simulink model "FaultModel"  (R2022b)
settings: Solver=VariableStepAuto  StartTime=0.0  StopTime=0.05  RelTol=1e-3
undefined symbols (not defined in the file or in its folder): D1, Delta
libraries: spsThreePhaseTransformerTwoWindingsLib x97, spsThreePhaseParallelRLCLoadLib x86, spsDistributedParametersLineLib x60, spsThreePhaseVIMeasurementLib x34, spsThreePhaseSourceLib x30, spsSeriesRLCBranchLib x3, spsGroundLib x2, spsCurrentMeasurementLib x1, spsThreePhaseFaultLib x1, spsVoltageMeasurementLib x1, spspowerguiLib x1
(part 4 of 4)

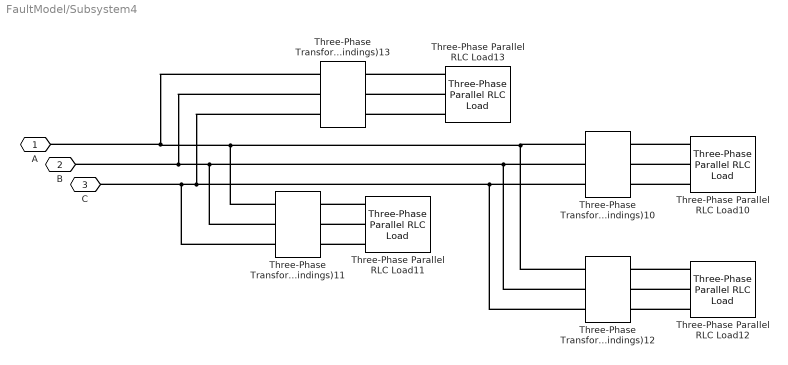
== system FaultModel/Subsystem4 ==
  Three-Phase Parallel RLC Load10 : spsThreePhaseParallelRLCLoadLib/Three-Phase Parallel RLC Load  LConnTagsString=A|B|C  Configuration=Y (grounded)  NominalVoltage=33e3  Vabc=[1e3 1e3 1e3]  Vabcp=[1e3 1e3 1e3]  NominalFrequency=50  UnbalancedPower=off  ActivePower=32.8e6  InductivePower=100  CapacitivePower=100  Pabc=[10e3 9e3 11e3]  QLabc=[100 90 110]  QCabc=[100 90 110]  Pabcp=[10e3 9e3 11e3]  QLabcp=[100 90 110]  QCabcp=[100 90 110]  Measurements=None  LoadType=constant Z
  Three-Phase Parallel RLC Load11 : spsThreePhaseParallelRLCLoadLib/Three-Phase Parallel RLC Load  LConnTagsString=A|B|C  Configuration=Y (grounded)  NominalVoltage=33e3  Vabc=[1e3 1e3 1e3]  Vabcp=[1e3 1e3 1e3]  NominalFrequency=50  UnbalancedPower=off  ActivePower=32.8e6  InductivePower=100  CapacitivePower=100  Pabc=[10e3 9e3 11e3]  QLabc=[100 90 110]  QCabc=[100 90 110]  Pabcp=[10e3 9e3 11e3]  QLabcp=[100 90 110]  QCabcp=[100 90 110]  Measurements=None  LoadType=constant Z
  Three-Phase Parallel RLC Load12 : spsThreePhaseParallelRLCLoadLib/Three-Phase Parallel RLC Load  LConnTagsString=A|B|C  Configuration=Y (grounded)  NominalVoltage=33e3  Vabc=[1e3 1e3 1e3]  Vabcp=[1e3 1e3 1e3]  NominalFrequency=50  UnbalancedPower=off  ActivePower=60e6  InductivePower=100  CapacitivePower=100  Pabc=[10e3 9e3 11e3]  QLabc=[100 90 110]  QCabc=[100 90 110]  Pabcp=[10e3 9e3 11e3]  QLabcp=[100 90 110]  QCabcp=[100 90 110]  Measurements=None  LoadType=constant Z
  Three-Phase Parallel RLC Load13 : spsThreePhaseParallelRLCLoadLib/Three-Phase Parallel RLC Load  LConnTagsString=A|B|C  Configuration=Y (grounded)  NominalVoltage=33e3  Vabc=[1e3 1e3 1e3]  Vabcp=[1e3 1e3 1e3]  NominalFrequency=50  UnbalancedPower=off  ActivePower=40e6  InductivePower=100  CapacitivePower=100  Pabc=[10e3 9e3 11e3]  QLabc=[100 90 110]  QCabc=[100 90 110]  Pabcp=[10e3 9e3 11e3]  QLabcp=[100 90 110]  QCabcp=[100 90 110]  Measurements=None  LoadType=constant Z
  Three-Phase Transformer (Two Windings)10 : spsThreePhaseTransformerTwoWindingsLib/Three-Phase Transformer (Two Windings)  Winding1Connection=Delta (D1)  Winding2Connection=Yg  CoreType=Three single-phase transformers  SetSaturation=off  Hysteresis=off  DataFile='hysteresis'  SetInitialFlux=off  Measurements=None  UNITS=pu  NominalPower=[ 41e6 , 50 ]  Winding1=[ 132e3 , 0.002 , 0.08 ]  Winding2=[ 33e3 , 0.002 , 0.08 ]  Rm=500  Lm=500  L0=0.5  Saturation=[ 0,0 ; 0.0024,1.2 ; 1.0,1.52 ]  InitialFluxes=[ 0.8 , -0.8 , 0.7 ]  BreakLoop=off  DiscreteSolver=Trapezoidal iterative  DataType=off  TransfoNumber=1
  Three-Phase Transformer (Two Windings)11 : spsThreePhaseTransformerTwoWindingsLib/Three-Phase Transformer (Two Windings)  Winding1Connection=Delta (D1)  Winding2Connection=Yg  CoreType=Three single-phase transformers  SetSaturation=off  Hysteresis=off  DataFile='hysteresis'  SetInitialFlux=off  Measurements=None  UNITS=pu  NominalPower=[ 41e6 , 50 ]  Winding1=[ 132e3 , 0.002 , 0.08 ]  Winding2=[ 33e3 , 0.002 , 0.08 ]  Rm=500  Lm=500  L0=0.5  Saturation=[ 0,0 ; 0.0024,1.2 ; 1.0,1.52 ]  InitialFluxes=[ 0.8 , -0.8 , 0.7 ]  BreakLoop=off  DiscreteSolver=Trapezoidal iterative  DataType=off  TransfoNumber=1
  Three-Phase Transformer (Two Windings)12 : spsThreePhaseTransformerTwoWindingsLib/Three-Phase Transformer (Two Windings)  Winding1Connection=Delta (D1)  Winding2Connection=Yg  CoreType=Three single-phase transformers  SetSaturation=off  Hysteresis=off  DataFile='hysteresis'  SetInitialFlux=off  Measurements=None  UNITS=pu  NominalPower=[ 75e6 , 50 ]  Winding1=[ 132e3 , 0.002 , 0.08 ]  Winding2=[ 33e3 , 0.002 , 0.08 ]  Rm=500  Lm=500  L0=0.5  Saturation=[ 0,0 ; 0.0024,1.2 ; 1.0,1.52 ]  InitialFluxes=[ 0.8 , -0.8 , 0.7 ]  BreakLoop=off  DiscreteSolver=Trapezoidal iterative  DataType=off  TransfoNumber=1
  Three-Phase Transformer (Two Windings)13 : spsThreePhaseTransformerTwoWindingsLib/Three-Phase Transformer (Two Windings)  Winding1Connection=Delta (D1)  Winding2Connection=Yg  CoreType=Three single-phase transformers  SetSaturation=off  Hysteresis=off  DataFile='hysteresis'  SetInitialFlux=off  Measurements=None  UNITS=pu  NominalPower=[50e6 , 50 ]  Winding1=[ 132e3 , 0.002 , 0.08 ]  Winding2=[ 33e3 , 0.002 , 0.08 ]  Rm=500  Lm=500  L0=0.5  Saturation=[ 0,0 ; 0.0024,1.2 ; 1.0,1.52 ]  InitialFluxes=[ 0.8 , -0.8 , 0.7 ]  BreakLoop=off  DiscreteSolver=Trapezoidal iterative  DataType=off  TransfoNumber=1
  A : PMIOPort  Side=Left
  B : PMIOPort  Port=2  Side=Left
  C : PMIOPort  Port=3  Side=Left
  connections:
  Three-Phase Parallel RLC Load10/LConn3 -- Three-Phase Transformer (Two Windings)10/RConn3
  Three-Phase Parallel RLC Load10/LConn2 -- Three-Phase Transformer (Two Windings)10/RConn2
  Three-Phase Parallel RLC Load13/LConn3 -- Three-Phase Transformer (Two Windings)13/RConn3
  Three-Phase Parallel RLC Load11/LConn3 -- Three-Phase Transformer (Two Windings)11/RConn3
  Three-Phase Transformer (Two Windings)13/LConn2 -- B/RConn1 -- Three-Phase Transformer (Two Windings)12/LConn2 -- Three-Phase Transformer (Two Windings)10/LConn2 -- Three-Phase Transformer (Two Windings)11/LConn2
  Three-Phase Parallel RLC Load12/LConn2 -- Three-Phase Transformer (Two Windings)12/RConn2
  Three-Phase Transformer (Two Windings)13/LConn1 -- Three-Phase Transformer (Two Windings)11/LConn1 -- Three-Phase Transformer (Two Windings)12/LConn1 -- Three-Phase Transformer (Two Windings)10/LConn1 -- A/RConn1
  Three-Phase Parallel RLC Load13/LConn2 -- Three-Phase Transformer (Two Windings)13/RConn2
  Three-Phase Parallel RLC Load12/LConn1 -- Three-Phase Transformer (Two Windings)12/RConn1
  Three-Phase Parallel RLC Load11/LConn2 -- Three-Phase Transformer (Two Windings)11/RConn2
  Three-Phase Parallel RLC Load11/LConn1 -- Three-Phase Transformer (Two Windings)11/RConn1
  Three-Phase Transformer (Two Windings)12/LConn3 -- C/RConn1 -- Three-Phase Transformer (Two Windings)11/LConn3 -- Three-Phase Transformer (Two Windings)13/LConn3 -- Three-Phase Transformer (Two Windings)10/LConn3
  Three-Phase Parallel RLC Load13/LConn1 -- Three-Phase Transformer (Two Windings)13/RConn1
  Three-Phase Parallel RLC Load12/LConn3 -- Three-Phase Transformer (Two Windings)12/RConn3
  Three-Phase Parallel RLC Load10/LConn1 -- Three-Phase Transformer (Two Windings)10/RConn1

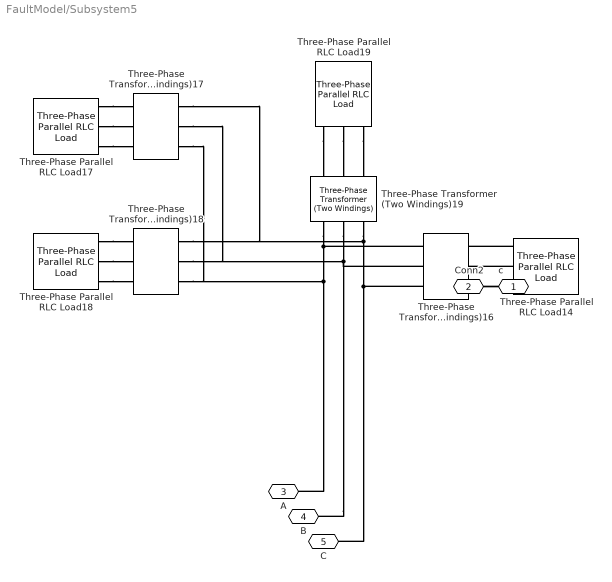
== system FaultModel/Subsystem5 ==
  Three-Phase Parallel RLC Load14 : spsThreePhaseParallelRLCLoadLib/Three-Phase Parallel RLC Load  LConnTagsString=A|B|C  Configuration=Y (grounded)  NominalVoltage=33e3  Vabc=[1e3 1e3 1e3]  Vabcp=[1e3 1e3 1e3]  NominalFrequency=50  UnbalancedPower=off  ActivePower=32.8e6  InductivePower=100  CapacitivePower=100  Pabc=[10e3 9e3 11e3]  QLabc=[100 90 110]  QCabc=[100 90 110]  Pabcp=[10e3 9e3 11e3]  QLabcp=[100 90 110]  QCabcp=[100 90 110]  Measurements=None  LoadType=constant Z
  Three-Phase Parallel RLC Load17 : spsThreePhaseParallelRLCLoadLib/Three-Phase Parallel RLC Load  LConnTagsString=A|B|C  Configuration=Y (grounded)  NominalVoltage=33e3  Vabc=[1e3 1e3 1e3]  Vabcp=[1e3 1e3 1e3]  NominalFrequency=50  UnbalancedPower=off  ActivePower=32.8e6  InductivePower=100  CapacitivePower=100  Pabc=[10e3 9e3 11e3]  QLabc=[100 90 110]  QCabc=[100 90 110]  Pabcp=[10e3 9e3 11e3]  QLabcp=[100 90 110]  QCabcp=[100 90 110]  Measurements=None  LoadType=constant Z
  Three-Phase Parallel RLC Load18 : spsThreePhaseParallelRLCLoadLib/Three-Phase Parallel RLC Load  LConnTagsString=A|B|C  Configuration=Y (grounded)  NominalVoltage=33e3  Vabc=[1e3 1e3 1e3]  Vabcp=[1e3 1e3 1e3]  NominalFrequency=50  UnbalancedPower=off  ActivePower=16e6  InductivePower=100  CapacitivePower=100  Pabc=[10e3 9e3 11e3]  QLabc=[100 90 110]  QCabc=[100 90 110]  Pabcp=[10e3 9e3 11e3]  QLabcp=[100 90 110]  QCabcp=[100 90 110]  Measurements=None  LoadType=constant Z
  Three-Phase Parallel RLC Load19 : spsThreePhaseParallelRLCLoadLib/Three-Phase Parallel RLC Load  LConnTagsString=A|B|C  Configuration=Y (grounded)  NominalVoltage=33e3  Vabc=[1e3 1e3 1e3]  Vabcp=[1e3 1e3 1e3]  NominalFrequency=50  UnbalancedPower=off  ActivePower=16e6  InductivePower=100  CapacitivePower=100  Pabc=[10e3 9e3 11e3]  QLabc=[100 90 110]  QCabc=[100 90 110]  Pabcp=[10e3 9e3 11e3]  QLabcp=[100 90 110]  QCabcp=[100 90 110]  Measurements=None  LoadType=constant Z
  Three-Phase Transformer (Two Windings)16 : spsThreePhaseTransformerTwoWindingsLib/Three-Phase Transformer (Two Windings)  Winding1Connection=Delta (D1)  Winding2Connection=Yg  CoreType=Three single-phase transformers  SetSaturation=off  Hysteresis=off  DataFile='hysteresis'  SetInitialFlux=off  Measurements=None  UNITS=pu  NominalPower=[41e6 , 50 ]  Winding1=[ 132e3 , 0.002 , 0.08 ]  Winding2=[ 33e3 , 0.002 , 0.08 ]  Rm=500  Lm=500  L0=0.5  Saturation=[ 0,0 ; 0.0024,1.2 ; 1.0,1.52 ]  InitialFluxes=[ 0.8 , -0.8 , 0.7 ]  BreakLoop=off  DiscreteSolver=Trapezoidal iterative  DataType=off  TransfoNumber=1
  Three-Phase Transformer (Two Windings)17 : spsThreePhaseTransformerTwoWindingsLib/Three-Phase Transformer (Two Windings)  Winding1Connection=Delta (D1)  Winding2Connection=Yg  CoreType=Three single-phase transformers  SetSaturation=off  Hysteresis=off  DataFile='hysteresis'  SetInitialFlux=off  Measurements=None  UNITS=pu  NominalPower=[41e6 , 50 ]  Winding1=[ 132e3 , 0.002 , 0.08 ]  Winding2=[ 33e3 , 0.002 , 0.08 ]  Rm=500  Lm=500  L0=0.5  Saturation=[ 0,0 ; 0.0024,1.2 ; 1.0,1.52 ]  InitialFluxes=[ 0.8 , -0.8 , 0.7 ]  BreakLoop=off  DiscreteSolver=Trapezoidal iterative  DataType=off  TransfoNumber=1
  Three-Phase Transformer (Two Windings)18 : spsThreePhaseTransformerTwoWindingsLib/Three-Phase Transformer (Two Windings)  Winding1Connection=Delta (D1)  Winding2Connection=Yg  CoreType=Three single-phase transformers  SetSaturation=off  Hysteresis=off  DataFile='hysteresis'  SetInitialFlux=off  Measurements=None  UNITS=pu  NominalPower=[20e6 , 50 ]  Winding1=[ 132e3 , 0.002 , 0.08 ]  Winding2=[ 33e3 , 0.002 , 0.08 ]  Rm=500  Lm=500  L0=0.5  Saturation=[ 0,0 ; 0.0024,1.2 ; 1.0,1.52 ]  InitialFluxes=[ 0.8 , -0.8 , 0.7 ]  BreakLoop=off  DiscreteSolver=Trapezoidal iterative  DataType=off  TransfoNumber=1
  Three-Phase Transformer (Two Windings)19 : spsThreePhaseTransformerTwoWindingsLib/Three-Phase Transformer (Two Windings)  Winding1Connection=Delta (D1)  Winding2Connection=Yg  CoreType=Three single-phase transformers  SetSaturation=off  Hysteresis=off  DataFile='hysteresis'  SetInitialFlux=off  Measurements=None  UNITS=pu  NominalPower=[20e6 , 50 ]  Winding1=[ 132e3 , 0.002 , 0.08 ]  Winding2=[ 33e3 , 0.002 , 0.08 ]  Rm=500  Lm=500  L0=0.5  Saturation=[ 0,0 ; 0.0024,1.2 ; 1.0,1.52 ]  InitialFluxes=[ 0.8 , -0.8 , 0.7 ]  BreakLoop=off  DiscreteSolver=Trapezoidal iterative  DataType=off  TransfoNumber=1
  c : PMIOPort  Side=Right
  Conn2 : PMIOPort  Port=2  Side=Left
  A : PMIOPort  Port=3  Side=Left
  B : PMIOPort  Port=4  Side=Left
  C : PMIOPort  Port=5  Side=Left
  connections:
  Three-Phase Transformer (Two Windings)19/LConn3 -- Three-Phase Transformer (Two Windings)17/LConn3 -- Three-Phase Transformer (Two Windings)18/LConn3 -- C/RConn1 -- Three-Phase Transformer (Two Windings)16/LConn3
  Three-Phase Transformer (Two Windings)19/LConn2 -- Three-Phase Transformer (Two Windings)17/LConn2 -- Three-Phase Transformer (Two Windings)18/LConn2 -- B/RConn1 -- Three-Phase Transformer (Two Windings)16/LConn2
  Three-Phase Transformer (Two Windings)19/LConn1 -- Three-Phase Transformer (Two Windings)16/LConn1 -- A/RConn1 -- Three-Phase Transformer (Two Windings)17/LConn1 -- Three-Phase Transformer (Two Windings)18/LConn1
  Three-Phase Parallel RLC Load17/LConn1 -- Three-Phase Transformer (Two Windings)17/RConn3
  Three-Phase Parallel RLC Load19/LConn1 -- Three-Phase Transformer (Two Windings)19/RConn1
  Three-Phase Parallel RLC Load14/LConn1 -- Three-Phase Transformer (Two Windings)16/RConn1
  Three-Phase Parallel RLC Load18/LConn2 -- Three-Phase Transformer (Two Windings)18/RConn2
  Three-Phase Parallel RLC Load17/LConn2 -- Three-Phase Transformer (Two Windings)17/RConn2
  Three-Phase Parallel RLC Load17/LConn3 -- Three-Phase Transformer (Two Windings)17/RConn1
  Three-Phase Parallel RLC Load19/LConn2 -- Three-Phase Transformer (Two Windings)19/RConn2
  Three-Phase Parallel RLC Load18/LConn1 -- Three-Phase Transformer (Two Windings)18/RConn3
  Three-Phase Parallel RLC Load19/LConn3 -- Three-Phase Transformer (Two Windings)19/RConn3
  Three-Phase Parallel RLC Load14/LConn2 -- Three-Phase Transformer (Two Windings)16/RConn2
  Three-Phase Parallel RLC Load18/LConn3 -- Three-Phase Transformer (Two Windings)18/RConn1
  Three-Phase Transformer (Two Windings)16/RConn3 -- c/RConn1
  Three-Phase Parallel RLC Load14/LConn3 -- Conn2/RConn1

== system FaultModel/Subsystem6 ==
  Three-Phase Parallel RLC Load20 : spsThreePhaseParallelRLCLoadLib/Three-Phase Parallel RLC Load  LConnTagsString=A|B|C  Configuration=Y (grounded)  NominalVoltage=33e3  Vabc=[1e3 1e3 1e3]  Vabcp=[1e3 1e3 1e3]  NominalFrequency=50  UnbalancedPower=off  ActivePower=32.8e6  InductivePower=100  CapacitivePower=100  Pabc=[10e3 9e3 11e3]  QLabc=[100 90 110]  QCabc=[100 90 110]  Pabcp=[10e3 9e3 11e3]  QLabcp=[100 90 110]  QCabcp=[100 90 110]  Measurements=None  LoadType=constant Z
  Three-Phase Parallel RLC Load21 : spsThreePhaseParallelRLCLoadLib/Three-Phase Parallel RLC Load  LConnTagsString=A|B|C  Configuration=Y (grounded)  NominalVoltage=33e3  Vabc=[1e3 1e3 1e3]  Vabcp=[1e3 1e3 1e3]  NominalFrequency=50  UnbalancedPower=off  ActivePower=32.8e6  InductivePower=100  CapacitivePower=100  Pabc=[10e3 9e3 11e3]  QLabc=[100 90 110]  QCabc=[100 90 110]  Pabcp=[10e3 9e3 11e3]  QLabcp=[100 90 110]  QCabcp=[100 90 110]  Measurements=None  LoadType=constant Z
  Three-Phase Parallel RLC Load22 : spsThreePhaseParallelRLCLoadLib/Three-Phase Parallel RLC Load  LConnTagsString=A|B|C  Configuration=Y (grounded)  NominalVoltage=33e3  Vabc=[1e3 1e3 1e3]  Vabcp=[1e3 1e3 1e3]  NominalFrequency=50  UnbalancedPower=off  ActivePower=32.8e6  InductivePower=100  CapacitivePower=100  Pabc=[10e3 9e3 11e3]  QLabc=[100 90 110]  QCabc=[100 90 110]  Pabcp=[10e3 9e3 11e3]  QLabcp=[100 90 110]  QCabcp=[100 90 110]  Measurements=None  LoadType=constant Z
  Three-Phase Transformer (Two Windings)20 : spsThreePhaseTransformerTwoWindingsLib/Three-Phase Transformer (Two Windings)  Winding1Connection=Delta (D1)  Winding2Connection=Yg  CoreType=Three single-phase transformers  SetSaturation=off  Hysteresis=off  DataFile='hysteresis'  SetInitialFlux=off  Measurements=None  UNITS=pu  NominalPower=[41e6 , 50 ]  Winding1=[ 132e3 , 0.002 , 0.08 ]  Winding2=[ 33e3 , 0.002 , 0.08 ]  Rm=500  Lm=500  L0=0.5  Saturation=[ 0,0 ; 0.0024,1.2 ; 1.0,1.52 ]  InitialFluxes=[ 0.8 , -0.8 , 0.7 ]  BreakLoop=off  DiscreteSolver=Trapezoidal iterative  DataType=off  TransfoNumber=1
  Three-Phase Transformer (Two Windings)21 : spsThreePhaseTransformerTwoWindingsLib/Three-Phase Transformer (Two Windings)  Winding1Connection=Delta (D1)  Winding2Connection=Yg  CoreType=Three single-phase transformers  SetSaturation=off  Hysteresis=off  DataFile='hysteresis'  SetInitialFlux=off  Measurements=None  UNITS=pu  NominalPower=[41e6 , 50 ]  Winding1=[ 132e3 , 0.002 , 0.08 ]  Winding2=[ 33e3 , 0.002 , 0.08 ]  Rm=500  Lm=500  L0=0.5  Saturation=[ 0,0 ; 0.0024,1.2 ; 1.0,1.52 ]  InitialFluxes=[ 0.8 , -0.8 , 0.7 ]  BreakLoop=off  DiscreteSolver=Trapezoidal iterative  DataType=off  TransfoNumber=1
  Three-Phase Transformer (Two Windings)22 : spsThreePhaseTransformerTwoWindingsLib/Three-Phase Transformer (Two Windings)  Winding1Connection=Delta (D1)  Winding2Connection=Yg  CoreType=Three single-phase transformers  SetSaturation=off  Hysteresis=off  DataFile='hysteresis'  SetInitialFlux=off  Measurements=None  UNITS=pu  NominalPower=[41e6 , 50 ]  Winding1=[ 132e3 , 0.002 , 0.08 ]  Winding2=[ 33e3 , 0.002 , 0.08 ]  Rm=500  Lm=500  L0=0.5  Saturation=[ 0,0 ; 0.0024,1.2 ; 1.0,1.52 ]  InitialFluxes=[ 0.8 , -0.8 , 0.7 ]  BreakLoop=off  DiscreteSolver=Trapezoidal iterative  DataType=off  TransfoNumber=1
  C : PMIOPort  Side=Left
  B : PMIOPort  Port=2  Side=Left
  A : PMIOPort  Port=3  Side=Left
  connections:
  Three-Phase Parallel RLC Load22/LConn2 -- Three-Phase Transformer (Two Windings)22/RConn2
  Three-Phase Parallel RLC Load22/LConn3 -- Three-Phase Transformer (Two Windings)22/RConn1
  Three-Phase Parallel RLC Load21/LConn2 -- Three-Phase Transformer (Two Windings)21/RConn2
  Three-Phase Parallel RLC Load20/LConn3 -- Three-Phase Transformer (Two Windings)20/RConn1
  Three-Phase Parallel RLC Load21/LConn3 -- Three-Phase Transformer (Two Windings)21/RConn1
  Three-Phase Parallel RLC Load21/LConn1 -- Three-Phase Transformer (Two Windings)21/RConn3
  Three-Phase Parallel RLC Load20/LConn2 -- Three-Phase Transformer (Two Windings)20/RConn2
  Three-Phase Parallel RLC Load20/LConn1 -- Three-Phase Transformer (Two Windings)20/RConn3
  Three-Phase Parallel RLC Load22/LConn1 -- Three-Phase Transformer (Two Windings)22/RConn3
  Three-Phase Transformer (Two Windings)22/LConn3 -- Three-Phase Transformer (Two Windings)21/LConn3 -- Three-Phase Transformer (Two Windings)20/LConn3 -- C/RConn1
  Three-Phase Transformer (Two Windings)22/LConn2 -- Three-Phase Transformer (Two Windings)20/LConn2 -- B/RConn1 -- Three-Phase Transformer (Two Windings)21/LConn2
  Three-Phase Transformer (Two Windings)22/LConn1 -- Three-Phase Transformer (Two Windings)21/LConn1 -- A/RConn1 -- Three-Phase Transformer (Two Windings)20/LConn1

== system FaultModel/Subsystem7 ==
  Three-Phase Parallel RLC Load23 : spsThreePhaseParallelRLCLoadLib/Three-Phase Parallel RLC Load  LConnTagsString=A|B|C  Configuration=Y (grounded)  NominalVoltage=33e3  Vabc=[1e3 1e3 1e3]  Vabcp=[1e3 1e3 1e3]  NominalFrequency=50  UnbalancedPower=off  ActivePower=60e6  InductivePower=100  CapacitivePower=100  Pabc=[10e3 9e3 11e3]  QLabc=[100 90 110]  QCabc=[100 90 110]  Pabcp=[10e3 9e3 11e3]  QLabcp=[100 90 110]  QCabcp=[100 90 110]  Measurements=None  LoadType=constant Z
  Three-Phase Parallel RLC Load24 : spsThreePhaseParallelRLCLoadLib/Three-Phase Parallel RLC Load  LConnTagsString=A|B|C  Configuration=Y (grounded)  NominalVoltage=33e3  Vabc=[1e3 1e3 1e3]  Vabcp=[1e3 1e3 1e3]  NominalFrequency=50  UnbalancedPower=off  ActivePower=60e6  InductivePower=100  CapacitivePower=100  Pabc=[10e3 9e3 11e3]  QLabc=[100 90 110]  QCabc=[100 90 110]  Pabcp=[10e3 9e3 11e3]  QLabcp=[100 90 110]  QCabcp=[100 90 110]  Measurements=None  LoadType=constant Z
  Three-Phase Transformer (Two Windings)23 : spsThreePhaseTransformerTwoWindingsLib/Three-Phase Transformer (Two Windings)  Winding1Connection=Delta (D1)  Winding2Connection=Yg  CoreType=Three single-phase transformers  SetSaturation=off  Hysteresis=off  DataFile='hysteresis'  SetInitialFlux=off  Measurements=None  UNITS=pu  NominalPower=[75e6 , 50 ]  Winding1=[ 132e3 , 0.002 , 0.08 ]  Winding2=[ 33e3 , 0.002 , 0.08 ]  Rm=500  Lm=500  L0=0.5  Saturation=[ 0,0 ; 0.0024,1.2 ; 1.0,1.52 ]  InitialFluxes=[ 0.8 , -0.8 , 0.7 ]  BreakLoop=off  DiscreteSolver=Trapezoidal iterative  DataType=off  TransfoNumber=1
  Three-Phase Transformer (Two Windings)24 : spsThreePhaseTransformerTwoWindingsLib/Three-Phase Transformer (Two Windings)  Winding1Connection=Delta (D1)  Winding2Connection=Yg  CoreType=Three single-phase transformers  SetSaturation=off  Hysteresis=off  DataFile='hysteresis'  SetInitialFlux=off  Measurements=None  UNITS=pu  NominalPower=[75e6 , 50 ]  Winding1=[ 132e3 , 0.002 , 0.08 ]  Winding2=[ 33e3 , 0.002 , 0.08 ]  Rm=500  Lm=500  L0=0.5  Saturation=[ 0,0 ; 0.0024,1.2 ; 1.0,1.52 ]  InitialFluxes=[ 0.8 , -0.8 , 0.7 ]  BreakLoop=off  DiscreteSolver=Trapezoidal iterative  DataType=off  TransfoNumber=1
  A : PMIOPort  Side=Left
  B : PMIOPort  Port=2  Side=Left
  C : PMIOPort  Port=3  Side=Left
  connections:
  Three-Phase Parallel RLC Load23/LConn2 -- Three-Phase Transformer (Two Windings)23/RConn2
  Three-Phase Parallel RLC Load23/LConn1 -- Three-Phase Transformer (Two Windings)23/RConn1
  Three-Phase Transformer (Two Windings)23/LConn2 -- B/RConn1 -- Three-Phase Transformer (Two Windings)24/LConn2
  Three-Phase Transformer (Two Windings)23/LConn3 -- C/RConn1 -- Three-Phase Transformer (Two Windings)24/LConn3
  Three-Phase Parallel RLC Load24/LConn3 -- Three-Phase Transformer (Two Windings)24/RConn3
  Three-Phase Transformer (Two Windings)23/LConn1 -- A/RConn1 -- Three-Phase Transformer (Two Windings)24/LConn1
  Three-Phase Parallel RLC Load23/LConn3 -- Three-Phase Transformer (Two Windings)23/RConn3
  Three-Phase Parallel RLC Load24/LConn2 -- Three-Phase Transformer (Two Windings)24/RConn2
  Three-Phase Parallel RLC Load24/LConn1 -- Three-Phase Transformer (Two Windings)24/RConn1

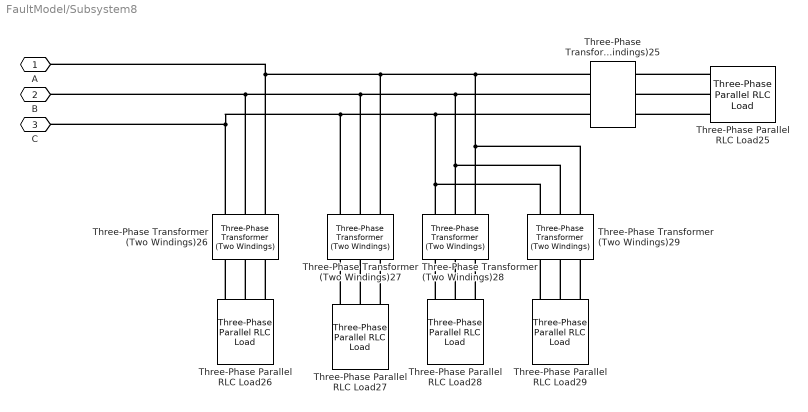
== system FaultModel/Subsystem8 ==
  Three-Phase Parallel RLC Load25 : spsThreePhaseParallelRLCLoadLib/Three-Phase Parallel RLC Load  LConnTagsString=A|B|C  Configuration=Y (grounded)  NominalVoltage=33e3  Vabc=[1e3 1e3 1e3]  Vabcp=[1e3 1e3 1e3]  NominalFrequency=50  UnbalancedPower=off  ActivePower=60e6  InductivePower=100  CapacitivePower=100  Pabc=[10e3 9e3 11e3]  QLabc=[100 90 110]  QCabc=[100 90 110]  Pabcp=[10e3 9e3 11e3]  QLabcp=[100 90 110]  QCabcp=[100 90 110]  Measurements=None  LoadType=constant Z
  Three-Phase Parallel RLC Load26 : spsThreePhaseParallelRLCLoadLib/Three-Phase Parallel RLC Load  LConnTagsString=A|B|C  Configuration=Y (grounded)  NominalVoltage=33e3  Vabc=[1e3 1e3 1e3]  Vabcp=[1e3 1e3 1e3]  NominalFrequency=50  UnbalancedPower=off  ActivePower=60e6  InductivePower=100  CapacitivePower=100  Pabc=[10e3 9e3 11e3]  QLabc=[100 90 110]  QCabc=[100 90 110]  Pabcp=[10e3 9e3 11e3]  QLabcp=[100 90 110]  QCabcp=[100 90 110]  Measurements=None  LoadType=constant Z
  Three-Phase Parallel RLC Load27 : spsThreePhaseParallelRLCLoadLib/Three-Phase Parallel RLC Load  LConnTagsString=A|B|C  Configuration=Y (grounded)  NominalVoltage=33e3  Vabc=[1e3 1e3 1e3]  Vabcp=[1e3 1e3 1e3]  NominalFrequency=50  UnbalancedPower=off  ActivePower=16e6  InductivePower=100  CapacitivePower=100  Pabc=[10e3 9e3 11e3]  QLabc=[100 90 110]  QCabc=[100 90 110]  Pabcp=[10e3 9e3 11e3]  QLabcp=[100 90 110]  QCabcp=[100 90 110]  Measurements=None  LoadType=constant Z
  Three-Phase Parallel RLC Load28 : spsThreePhaseParallelRLCLoadLib/Three-Phase Parallel RLC Load  LConnTagsString=A|B|C  Configuration=Y (grounded)  NominalVoltage=33e3  Vabc=[1e3 1e3 1e3]  Vabcp=[1e3 1e3 1e3]  NominalFrequency=50  UnbalancedPower=off  ActivePower=16e6  InductivePower=100  CapacitivePower=100  Pabc=[10e3 9e3 11e3]  QLabc=[100 90 110]  QCabc=[100 90 110]  Pabcp=[10e3 9e3 11e3]  QLabcp=[100 90 110]  QCabcp=[100 90 110]  Measurements=None  LoadType=constant Z
  Three-Phase Parallel RLC Load29 : spsThreePhaseParallelRLCLoadLib/Three-Phase Parallel RLC Load  LConnTagsString=A|B|C  Configuration=Y (grounded)  NominalVoltage=33e3  Vabc=[1e3 1e3 1e3]  Vabcp=[1e3 1e3 1e3]  NominalFrequency=50  UnbalancedPower=off  ActivePower=26.4e6  InductivePower=100  CapacitivePower=100  Pabc=[10e3 9e3 11e3]  QLabc=[100 90 110]  QCabc=[100 90 110]  Pabcp=[10e3 9e3 11e3]  QLabcp=[100 90 110]  QCabcp=[100 90 110]  Measurements=None  LoadType=constant Z
  Three-Phase Transformer (Two Windings)25 : spsThreePhaseTransformerTwoWindingsLib/Three-Phase Transformer (Two Windings)  Winding1Connection=Delta (D1)  Winding2Connection=Yg  CoreType=Three single-phase transformers  SetSaturation=off  Hysteresis=off  DataFile='hysteresis'  SetInitialFlux=off  Measurements=None  UNITS=pu  NominalPower=[75e6 , 50 ]  Winding1=[ 132e3 , 0.002 , 0.08 ]  Winding2=[ 33e3 , 0.002 , 0.08 ]  Rm=500  Lm=500  L0=0.5  Saturation=[ 0,0 ; 0.0024,1.2 ; 1.0,1.52 ]  InitialFluxes=[ 0.8 , -0.8 , 0.7 ]  BreakLoop=off  DiscreteSolver=Trapezoidal iterative  DataType=off  TransfoNumber=1
  Three-Phase Transformer (Two Windings)26 : spsThreePhaseTransformerTwoWindingsLib/Three-Phase Transformer (Two Windings)  Winding1Connection=Delta (D1)  Winding2Connection=Yg  CoreType=Three single-phase transformers  SetSaturation=off  Hysteresis=off  DataFile='hysteresis'  SetInitialFlux=off  Measurements=None  UNITS=pu  NominalPower=[75e6 , 50 ]  Winding1=[ 132e3 , 0.002 , 0.08 ]  Winding2=[ 33e3 , 0.002 , 0.08 ]  Rm=500  Lm=500  L0=0.5  Saturation=[ 0,0 ; 0.0024,1.2 ; 1.0,1.52 ]  InitialFluxes=[ 0.8 , -0.8 , 0.7 ]  BreakLoop=off  DiscreteSolver=Trapezoidal iterative  DataType=off  TransfoNumber=1
  Three-Phase Transformer (Two Windings)27 : spsThreePhaseTransformerTwoWindingsLib/Three-Phase Transformer (Two Windings)  Winding1Connection=Delta (D1)  Winding2Connection=Yg  CoreType=Three single-phase transformers  SetSaturation=off  Hysteresis=off  DataFile='hysteresis'  SetInitialFlux=off  Measurements=None  UNITS=pu  NominalPower=[20e6 , 50 ]  Winding1=[ 132e3 , 0.002 , 0.08 ]  Winding2=[ 33e3 , 0.002 , 0.08 ]  Rm=500  Lm=500  L0=0.5  Saturation=[ 0,0 ; 0.0024,1.2 ; 1.0,1.52 ]  InitialFluxes=[ 0.8 , -0.8 , 0.7 ]  BreakLoop=off  DiscreteSolver=Trapezoidal iterative  DataType=off  TransfoNumber=1
  Three-Phase Transformer (Two Windings)28 : spsThreePhaseTransformerTwoWindingsLib/Three-Phase Transformer (Two Windings)  Winding1Connection=Delta (D1)  Winding2Connection=Yg  CoreType=Three single-phase transformers  SetSaturation=off  Hysteresis=off  DataFile='hysteresis'  SetInitialFlux=off  Measurements=None  UNITS=pu  NominalPower=[20e6 , 50 ]  Winding1=[ 132e3 , 0.002 , 0.08 ]  Winding2=[ 33e3 , 0.002 , 0.08 ]  Rm=500  Lm=500  L0=0.5  Saturation=[ 0,0 ; 0.0024,1.2 ; 1.0,1.52 ]  InitialFluxes=[ 0.8 , -0.8 , 0.7 ]  BreakLoop=off  DiscreteSolver=Trapezoidal iterative  DataType=off  TransfoNumber=1
  Three-Phase Transformer (Two Windings)29 : spsThreePhaseTransformerTwoWindingsLib/Three-Phase Transformer (Two Windings)  Winding1Connection=Delta (D1)  Winding2Connection=Yg  CoreType=Three single-phase transformers  SetSaturation=off  Hysteresis=off  DataFile='hysteresis'  SetInitialFlux=off  Measurements=None  UNITS=pu  NominalPower=[33e6 , 50 ]  Winding1=[ 132e3 , 0.002 , 0.08 ]  Winding2=[ 33e3 , 0.002 , 0.08 ]  Rm=500  Lm=500  L0=0.5  Saturation=[ 0,0 ; 0.0024,1.2 ; 1.0,1.52 ]  InitialFluxes=[ 0.8 , -0.8 , 0.7 ]  BreakLoop=off  DiscreteSolver=Trapezoidal iterative  DataType=off  TransfoNumber=1
  A : PMIOPort  Side=Left
  B : PMIOPort  Port=2  Side=Left
  C : PMIOPort  Port=3  Side=Left
  connections:
  Three-Phase Transformer (Two Windings)25/LConn2 -- Three-Phase Transformer (Two Windings)28/LConn2 -- Three-Phase Transformer (Two Windings)29/LConn2 -- Three-Phase Transformer (Two Windings)27/LConn2 -- B/RConn1 -- Three-Phase Transformer (Two Windings)26/LConn2
  Three-Phase Parallel RLC Load25/LConn2 -- Three-Phase Transformer (Two Windings)25/RConn2
  Three-Phase Parallel RLC Load29/LConn3 -- Three-Phase Transformer (Two Windings)29/RConn1
  Three-Phase Parallel RLC Load28/LConn2 -- Three-Phase Transformer (Two Windings)28/RConn2
  Three-Phase Parallel RLC Load25/LConn3 -- Three-Phase Transformer (Two Windings)25/RConn3
  Three-Phase Transformer (Two Windings)25/LConn3 -- Three-Phase Transformer (Two Windings)29/LConn3 -- Three-Phase Transformer (Two Windings)28/LConn3 -- Three-Phase Transformer (Two Windings)26/LConn3 -- C/RConn1 -- Three-Phase Transformer (Two Windings)27/LConn3
  Three-Phase Parallel RLC Load27/LConn1 -- Three-Phase Transformer (Two Windings)27/RConn3
  Three-Phase Transformer (Two Windings)25/LConn1 -- Three-Phase Transformer (Two Windings)28/LConn1 -- Three-Phase Transformer (Two Windings)29/LConn1 -- Three-Phase Transformer (Two Windings)27/LConn1 -- A/RConn1 -- Three-Phase Transformer (Two Windings)26/LConn1
  Three-Phase Parallel RLC Load28/LConn3 -- Three-Phase Transformer (Two Windings)28/RConn1
  Three-Phase Parallel RLC Load29/LConn2 -- Three-Phase Transformer (Two Windings)29/RConn2
  Three-Phase Parallel RLC Load26/LConn2 -- Three-Phase Transformer (Two Windings)26/RConn2
  Three-Phase Parallel RLC Load26/LConn1 -- Three-Phase Transformer (Two Windings)26/RConn3
  Three-Phase Parallel RLC Load28/LConn1 -- Three-Phase Transformer (Two Windings)28/RConn3
  Three-Phase Parallel RLC Load27/LConn2 -- Three-Phase Transformer (Two Windings)27/RConn2
  Three-Phase Parallel RLC Load29/LConn1 -- Three-Phase Transformer (Two Windings)29/RConn3
  Three-Phase Parallel RLC Load27/LConn3 -- Three-Phase Transformer (Two Windings)27/RConn1
  Three-Phase Parallel RLC Load25/LConn1 -- Three-Phase Transformer (Two Windings)25/RConn1
  Three-Phase Parallel RLC Load26/LConn3 -- Three-Phase Transformer (Two Windings)26/RConn1

== system FaultModel/Subsystem9 ==
  Three-Phase Parallel RLC Load{30..33} (4 alike) : spsThreePhaseParallelRLCLoadLib/Three-Phase Parallel RLC Load  LConnTagsString=A|B|C  Configuration=Y (grounded)  NominalVoltage=33e3  Vabc=[1e3 1e3 1e3]  Vabcp=[1e3 1e3 1e3]  NominalFrequency=50  UnbalancedPower=off  ActivePower=10e3  InductivePower=100  CapacitivePower=100  Pabc=[10e3 9e3 11e3]  QLabc=[100 90 110]  QCabc=[100 90 110]  Pabcp=[10e3 9e3 11e3]  QLabcp=[100 90 110]  QCabcp=[100 90 110]  Measurements=None  LoadType=constant Z
  Three-Phase Transformer (Two Windings)30 : spsThreePhaseTransformerTwoWindingsLib/Three-Phase Transformer (Two Windings)  Winding1Connection=Delta (D1)  Winding2Connection=Yg  CoreType=Three single-phase transformers  SetSaturation=off  Hysteresis=off  DataFile='hysteresis'  SetInitialFlux=off  Measurements=None  UNITS=pu  NominalPower=[41e6 , 50 ]  Winding1=[ 132e3 , 0.002 , 0.08 ]  Winding2=[ 33e3 , 0.002 , 0.08 ]  Rm=500  Lm=500  L0=0.5  Saturation=[ 0,0 ; 0.0024,1.2 ; 1.0,1.52 ]  InitialFluxes=[ 0.8 , -0.8 , 0.7 ]  BreakLoop=off  DiscreteSolver=Trapezoidal iterative  DataType=off  TransfoNumber=1
  Three-Phase Transformer (Two Windings)31 : spsThreePhaseTransformerTwoWindingsLib/Three-Phase Transformer (Two Windings)  Winding1Connection=Delta (D1)  Winding2Connection=Yg  CoreType=Three single-phase transformers  SetSaturation=off  Hysteresis=off  DataFile='hysteresis'  SetInitialFlux=off  Measurements=None  UNITS=pu  NominalPower=[41e6 , 50 ]  Winding1=[ 132e3 , 0.002 , 0.08 ]  Winding2=[ 33e3 , 0.002 , 0.08 ]  Rm=500  Lm=500  L0=0.5  Saturation=[ 0,0 ; 0.0024,1.2 ; 1.0,1.52 ]  InitialFluxes=[ 0.8 , -0.8 , 0.7 ]  BreakLoop=off  DiscreteSolver=Trapezoidal iterative  DataType=off  TransfoNumber=1
  Three-Phase Transformer (Two Windings)32 : spsThreePhaseTransformerTwoWindingsLib/Three-Phase Transformer (Two Windings)  Winding1Connection=Delta (D1)  Winding2Connection=Yg  CoreType=Three single-phase transformers  SetSaturation=off  Hysteresis=off  DataFile='hysteresis'  SetInitialFlux=off  Measurements=None  UNITS=pu  NominalPower=[75e6 , 50 ]  Winding1=[ 132e3 , 0.002 , 0.08 ]  Winding2=[ 33e3 , 0.002 , 0.08 ]  Rm=500  Lm=500  L0=0.5  Saturation=[ 0,0 ; 0.0024,1.2 ; 1.0,1.52 ]  InitialFluxes=[ 0.8 , -0.8 , 0.7 ]  BreakLoop=off  DiscreteSolver=Trapezoidal iterative  DataType=off  TransfoNumber=1
  Three-Phase Transformer (Two Windings)33 : spsThreePhaseTransformerTwoWindingsLib/Three-Phase Transformer (Two Windings)  Winding1Connection=Delta (D1)  Winding2Connection=Yg  CoreType=Three single-phase transformers  SetSaturation=off  Hysteresis=off  DataFile='hysteresis'  SetInitialFlux=off  Measurements=None  UNITS=pu  NominalPower=[75e6 , 50 ]  Winding1=[ 132e3 , 0.002 , 0.08 ]  Winding2=[ 33e3 , 0.002 , 0.08 ]  Rm=500  Lm=500  L0=0.5  Saturation=[ 0,0 ; 0.0024,1.2 ; 1.0,1.52 ]  InitialFluxes=[ 0.8 , -0.8 , 0.7 ]  BreakLoop=off  DiscreteSolver=Trapezoidal iterative  DataType=off  TransfoNumber=1
  A : PMIOPort  Side=Left
  B : PMIOPort  Port=2  Side=Left
  C : PMIOPort  Port=3  Side=Left
  connections:
  Three-Phase Parallel RLC Load33/LConn3 -- Three-Phase Transformer (Two Windings)33/RConn3
  Three-Phase Parallel RLC Load30/LConn2 -- Three-Phase Transformer (Two Windings)30/RConn2
  Three-Phase Parallel RLC Load31/LConn3 -- Three-Phase Transformer (Two Windings)31/RConn3
  Three-Phase Transformer (Two Windings)32/LConn1 -- Three-Phase Transformer (Two Windings)30/LConn1 -- A/RConn1 -- Three-Phase Transformer (Two Windings)33/LConn1 -- Three-Phase Transformer (Two Windings)31/LConn1
  Three-Phase Parallel RLC Load32/LConn3 -- Three-Phase Transformer (Two Windings)32/RConn3
  Three-Phase Parallel RLC Load32/LConn1 -- Three-Phase Transformer (Two Windings)32/RConn1
  Three-Phase Transformer (Two Windings)30/LConn3 -- C/RConn1 -- Three-Phase Transformer (Two Windings)33/LConn3 -- Three-Phase Transformer (Two Windings)31/LConn3 -- Three-Phase Transformer (Two Windings)32/LConn3
  Three-Phase Transformer (Two Windings)32/LConn2 -- Three-Phase Transformer (Two Windings)30/LConn2 -- B/RConn1 -- Three-Phase Transformer (Two Windings)33/LConn2 -- Three-Phase Transformer (Two Windings)31/LConn2
  Three-Phase Parallel RLC Load33/LConn2 -- Three-Phase Transformer (Two Windings)33/RConn2
  Three-Phase Parallel RLC Load31/LConn2 -- Three-Phase Transformer (Two Windings)31/RConn2
  Three-Phase Parallel RLC Load33/LConn1 -- Three-Phase Transformer (Two Windings)33/RConn1
  Three-Phase Parallel RLC Load31/LConn1 -- Three-Phase Transformer (Two Windings)31/RConn1
  Three-Phase Parallel RLC Load32/LConn2 -- Three-Phase Transformer (Two Windings)32/RConn2
  Three-Phase Parallel RLC Load30/LConn1 -- Three-Phase Transformer (Two Windings)30/RConn1
  Three-Phase Parallel RLC Load30/LConn3 -- Three-Phase Transformer (Two Windings)30/RConn3
